simulink model "lab8symu"  (R2023b)
settings: Solver=VariableStepAuto  StartTime=0.0  StopTime=time  RelTol=1e-3
values from neighbouring files (symbols this model uses):
  a = -2    [lab8.m]    (also in skrypt_TS_Lab_8a.m = -1)
  A = 1.5    [lab8.m]
  Au = 5    [lab8.m]
  b = 2    [lab8.m]    (also in skrypt_TS_Lab_8a.m = 1)
  c = 1    [lab8.m]    (also in skrypt_TS_Lab_8a.m)
  const = 3    [lab8.m]
  f = 100    [lab8.m]
  fu = 0.05    [lab8.m]
  licznik = Ko.num{1}    [lab8.m]
  mianownik = Ko.den{1}    [lab8.m]
settings Model: Creator=pc  LastModifiedBy=pc

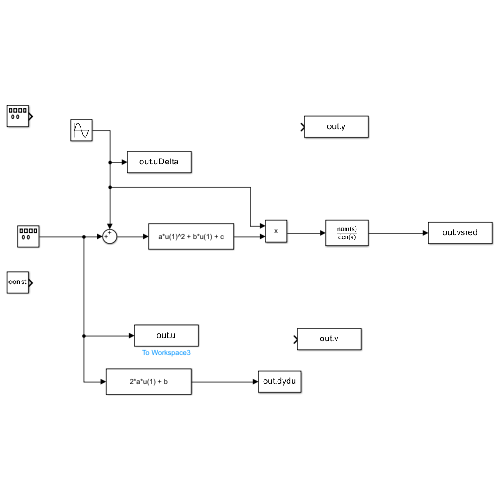
[thumbnail: Simulink's stored preview of the top-level diagram]
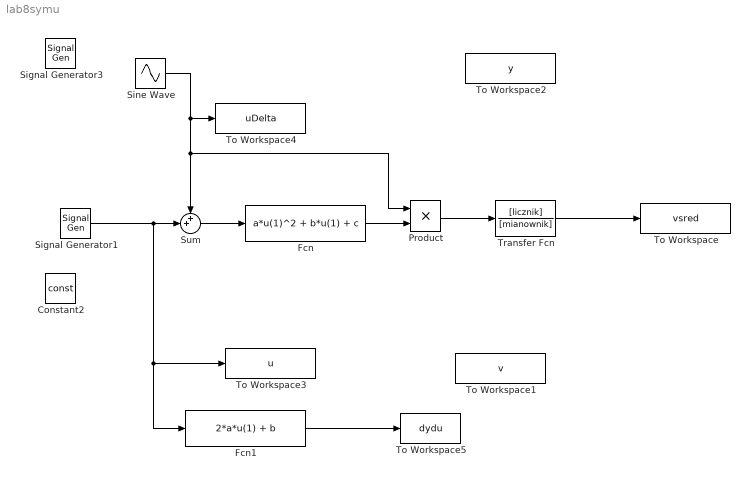
== system lab8symu ==
  Constant2 : Constant  Value=const
  Fcn : Fcn  Expr=a*u(1)^2 + b*u(1) + c
  Fcn1 : Fcn  Expr=2*a*u(1) + b
  Product : Product
  Signal Generator1 : SignalGenerator  WaveForm=square  Amplitude=Au  Frequency=fu
  Signal Generator3 : SignalGenerator  Amplitude=A  Frequency=f
  Sine Wave : Sin  Amplitude=A  Frequency=f  SampleTime=0
  Sum : Sum  Inputs=++|
  To Workspace : ToWorkspace  VariableName=vsred  SaveFormat=Timeseries  SampleTime=-1
  To Workspace1 : ToWorkspace  VariableName=v  SaveFormat=Timeseries  SampleTime=-1
  To Workspace2 : ToWorkspace  VariableName=y  SaveFormat=Timeseries  SampleTime=-1
  To Workspace3 : ToWorkspace  VariableName=u  SaveFormat=Timeseries  SampleTime=-1
  To Workspace4 : ToWorkspace  VariableName=uDelta  SaveFormat=Timeseries  SampleTime=-1
  To Workspace5 : ToWorkspace  VariableName=dydu  SampleTime=-1
  Transfer Fcn : TransferFcn  Numerator=[licznik]  Denominator=[mianownik]
  wires:
  Sum/1 -> Fcn/1
  Signal Generator1/1 -> Fcn1/1, To Workspace3/1, Sum/2
  Sine Wave/1 -> To Workspace4/1, Product/1, Sum/1
  Fcn/1 -> Product/2
  Product/1 -> Transfer Fcn/1
  Transfer Fcn/1 -> To Workspace/1
  Fcn1/1 -> To Workspace5/1
